simulink model "Approach_Avoid_Task"  (R2019b)
settings: Solver=ode4  StartTime=0.0  StopTime=inf  FixedStep=BKIN_STEP_TIME  RelTol=1e-3  EnableMultiTasking=on
StartFcn:
  |  warndlg('Dexterit-E models cannot run under simulation. Please compile your model and run it from within Dexterit-E.');set_param(bdroot,'SimulationCommand','stop')
model workspace (MAT data in the model file):
  ADJUST_START = 2
  APPROACH_TARGET_COL = 9
  AVOIDVIS_AREA_COL = 3
  AVOID_AREA_COL = 2
  AVOID_DIST_ADJUST = 8
  BEGIN_LABEL_COL = 5
  BEGIN_TARGET_COL = 4
  BKIN_KINEMATIC_FRAME_SIZE = 400
  BKIN_STEP_TIME = 0.00025
  CHECK_ORDER_ACTIVE = 7
  CHECK_ORDER_CIRC = 6
  COLOUR_2ND = 7
  COLOUR_3RD = 11
  COLOUR_4TH = 12
  COLOUR_INIT = 6
  ERROR_DELAY = 12
  ERROR_LABEL_COL = 6
  E_APPROACHED = 19
  E_AVOIDED = 21
  E_BLOCK_1 = 28
  E_BLOCK_2 = 29
  E_BLOCK_3 = 30
  E_BLOCK_4 = 31
  E_ERROR_TRIAL = 23
  E_HAND_IN_START = 17
  E_HAND_LEFT = 16
  E_LEFT_TESTED = 2
  E_LOC_1 = 3
  E_LOC_10 = 12
  E_LOC_11 = 13
  E_LOC_12 = 14
  E_LOC_2 = 4
  E_LOC_3 = 5
  E_LOC_4 = 6
  E_LOC_5 = 7
  E_LOC_6 = 8
  E_LOC_7 = 9
  E_LOC_8 = 10
  E_LOC_9 = 11
  E_NO_EVENT = 0
  E_RIGHT_TESTED = 1
  E_TARGET_ON = 18
  E_TASK_SEQ_1 = 24
  E_TASK_SEQ_2 = 25
  E_TASK_SEQ_3 = 26
  E_TASK_SEQ_4 = 27
  E_TIMED_OUT = 22
  E_TRIAL_END = 20
  E_TRIAL_START = 15
  INFO_TARGET_COL = 8
  LABEL_HEIGHT = 9
  LABEL_TEXT = 8
  LENGTH = 3
  MAX_FORCE = 3
  MAX_FORCE_BG = 4
  NO_SANDWICH = 15
  RADIUS_VIS = 3
  RAMP_DURATION = 5
  RAND_START_DELAY = 10
  REACH_TIME = 13
  SLOW_LABEL_COL = 7
  START_HOLD_DELAY = 9
  START_TARGET_COL = 1
  STROKE_WIDTH = 10
  SUCCESS_DELAY = 11
  TARGET_X = 4
  TARGET_Y = 5
  TARG_DIST = 1
  TARG_LENGTH = 3
  TARG_WIDTH = 4
  TOGGLE_FIELD = 10
  TRIAL_TIME = 14
  WIDTH = 4
  Width = 4
  col_x = 1
  col_y = 2
undefined symbols (not defined in the file): slselsubs
libraries: Video x10, KINARM_EP_loads x5, General x3, KINARM_general x3
settings Model: ModifiedComment=chris -- Wed Feb 16 09:18:30 2005 -- Version 1.1384  ModifiedHistory=Feb 16/05 - Add error repeat, add offset ramp  ExtModeArmWhenConnect=off  ExtModeLogAll=off  OrderedModelArguments=off  Creator=Chris Grebeldinger  LastModifiedBy=User
settings SolverCC: AutoInsertRateTranBlk=on
settings DataIOCC: SaveFormat=Array  SignalLoggingSaveFormat=ModelDataLogs  SaveOutput=off  SaveTime=off  ReturnWorkspaceOutputs=off  SignalLoggingName=sigsOut
settings OptimizationCC: BlockReduction=off  BooleanDataType=off  OptimizeBlockIOStorage=off  BufferReuse=off  GlobalBufferReuse=off  ExpressionFolding=off  ExpressionDepthLimit=2147483647  LocalBlockOutputs=off  InitFltsAndDblsToZero=on  LifeSpan=inf  OptimizeDataStoreBuffers=off  BusAssignmentInplaceUpdate=off
settings DebuggingCC: SaveWithParameterizedLinksMsg=none  UnderspecifiedInitializationDetection=Classic  MergeDetectMultiDrivingBlocksExec=none  SignalResolutionControl=TryResolveAllWithWarning  MultiTaskDSMMsg=warning  FcnCallInpInsideContextMsg=warning  BusObjectLabelMismatch=none  StateNameClashWarn=warning  StrictBusMsg=ErrorOnBusTreatedAsVector  SFUnexpectedBacktrackingDiag=warning  SFNoUnconditionalDefaultTransitionDiag=warning  SFExecutionAtInitializationDiag=none  ArithmeticOperatorsInVariantConditions=warning
settings HardwareCC: ProdBitPerPointer=32  ProdBitPerSizeT=32  ProdBitPerPtrDiffT=32  ProdLargestAtomicFloat=None  ProdWordSize=32  ProdLongLongMode=on  ProdHWDeviceType=Generic->32-bit x86 compatible  TargetLongLongMode=on  TargetIntDivRoundTo=Zero  TargetEndianess=LittleEndian  TargetHWDeviceType=Generic->32-bit x86 compatible
settings ModelReferenceCC: PropagateSignalLabelsOutOfModel=off
settings SFSimCC: SimCustomHeaderCode="#include \"stdlib.h\""  SimUseLocalCustomCode=off  SimParseCustomCode=off  CustomCodeUndefinedFunction=UseInterfaceOnly
settings RTWCC: Description=Simulink Real-Time  SystemTargetFile=slrt.tlc  TemplateMakefile=slrt_default_tmf  RTWUseLocalCustomCode=off  CustomSourceCode="#include \"stdlib.h\""  CodeExecutionProfiling=on
settings CodeAppCC: MaxIdLength=63  StateflowObjectComments=on
settings SimulinkRealTimeCC: TargetFcnLib=ansi_tfl_tmw.mat  GeneratePreprocessorConditionals=Disable all  PreserveStateflowLocalDataDimensions=off
settings ConfigComp: CovMetricSettings=dw  CovHtmlReporting=on  CovSaveCumulativeToWorkspaceVar=on  CovSaveSingleToWorkspaceVar=on  CovExternalEMLEnable=off

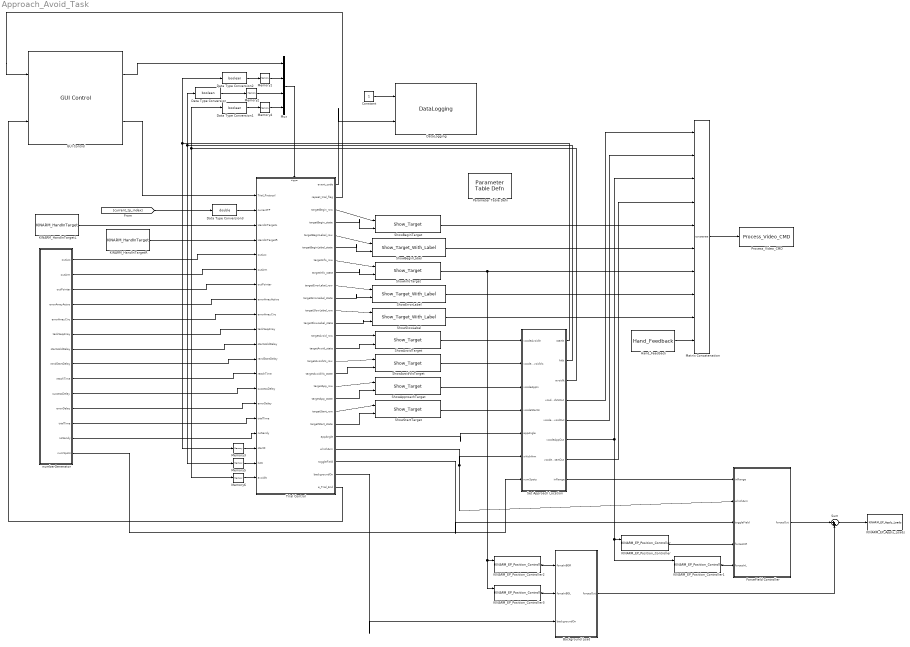
== system Approach_Avoid_Task ==
  Background Load : Subsystem
  Constant : Constant
  Data Type Conversion : DataTypeConversion  OutDataTypeStr=boolean
  Data Type Conversion1 : DataTypeConversion  OutDataTypeStr=boolean
  Data Type Conversion2 : DataTypeConversion  OutDataTypeStr=boolean
  Data Type Conversion3 : DataTypeConversion  OutDataTypeStr=double
  DataLogging : General/DataLogging  log_event_codes=on  log_analog_inputs=off  show_time_remaining=off  ecat_include=on
  ForceField Controller : Subsystem
  GUI Control : General/GUI Control  task_version=1.0  show_repeat_trial_flag=on  use_custom_tp=off  target_type_str=Circle  Target_Type=1  XYcols=[1 2]  Vcols=3  Lcols=4  indices_padding=[0 0 0 0;0 0 0 0]  target_table_rows=64  load_table_rows=20  tp_table_rows=100
  Hand_Feedback : KINARM_general/Hand_Feedback  feedback_cntl_src=none
  KINARM_EP_Apply_Loads : KINARM_EP_loads/KINARM_EP_Apply_Loads  up_duration=1500  down_duration=1500  max_force=30
  KINARM_EP_Position_Controller : KINARM_EP_loads/KINARM_EP_Position_Controller  use_dom_hand=on  inertias_for_FF=KINARM End Point robot  gain_choice=Standard Movement  sample_time=0.001
  KINARM_EP_Position_Controller1 : KINARM_EP_loads/KINARM_EP_Position_Controller  use_dom_hand=off  inertias_for_FF=KINARM End Point robot  gain_choice=Standard Movement  sample_time=0.001
  KINARM_EP_Position_Controller2 : KINARM_EP_loads/KINARM_EP_Position_Controller  use_dom_hand=on  inertias_for_FF=KINARM End Point robot  gain_choice=Standard Movement  sample_time=0.001
  KINARM_EP_Position_Controller3 : KINARM_EP_loads/KINARM_EP_Position_Controller  use_dom_hand=off  inertias_for_FF=KINARM End Point robot  gain_choice=Standard Movement  sample_time=0.001
  KINARM_HandInTargetL : KINARM_general/KINARM_HandInTarget  use_dominant_hand=off  target_type=Circle  num_states=1  attribcol1=[RADIUS_VIS]  attribcol2=[0]  attribcol3=[0]  attribcol4=[0]  attribcol5=[0]
  KINARM_HandInTargetR : KINARM_general/KINARM_HandInTarget  use_dominant_hand=on  target_type=Circle  num_states=1  attribcol1=[RADIUS_VIS]  attribcol2=[0]  attribcol3=[0]  attribcol4=[0]  attribcol5=[0]
  Matrix Concatenation : Concatenate  NumInputs=10  Mode=Multidimensional array
  Memory{1..6} (6 alike) : Memory
  Mux : Mux
  Parameter Table Defn : General/Parameter Table Defn  ShowInLibBrowser=0
  Process_Video_CMD : Video/Process_Video_CMD  video_delay=50
  Set Approach Location : Subsystem
  ShowApproachTarget : Video/Show_Target  target_type=Circle  num_states=1  attribcol1=[COLOUR_INIT 0 0 RADIUS_VIS]  attribcol2=[0 0 0 0]  attribcol3=[0 0 0 0]  attribcol4=[0 0 0 0]  attribcol5=[0 0 0 0]  stateindices_padding=[0 0 0 0 0 0 0;0 0 0 0 0 0 0;0 0 0 0 0 0 0;0 0 0 0 0 0 0;0 0 0 0 0 0 0]  source=dialog  opacity=100  target_display=Both subject and operator displays  num_col=4
  ShowAvoidTarget : Video/Show_Target  target_type=Circle  num_states=1  attribcol1=[COLOUR_INIT COLOUR_2ND STROKE_WIDTH RADIUS_VIS]  attribcol2=[0 0 0 0]  attribcol3=[0 0 0 0]  attribcol4=[0 0 0 0]  attribcol5=[0 0 0 0]  stateindices_padding=[0 0 0 0 0 0 0;0 0 0 0 0 0 0;0 0 0 0 0 0 0;0 0 0 0 0 0 0;0 0 0 0 0 0 0]  source=dialog  opacity=100  target_display=Both subject and operator displays  num_col=4
  ShowAvoidVisTarget : Video/Show_Target  target_type=Circle  num_states=1  attribcol1=[COLOUR_INIT COLOUR_2ND STROKE_WIDTH RADIUS_VIS]  attribcol2=[0 0 0 0]  attribcol3=[0 0 0 0]  attribcol4=[0 0 0 0]  attribcol5=[0 0 0 0]  stateindices_padding=[0 0 0 0 0 0 0;0 0 0 0 0 0 0;0 0 0 0 0 0 0;0 0 0 0 0 0 0;0 0 0 0 0 0 0]  source=dialog  opacity=100  target_display=Both subject and operator displays  num_col=4
  ShowBeginLabel : Video/Show_Target_With_Label  target_type=Circle  num_states=1  attribcol1=[0 0 0 0 LABEL_TEXT COLOUR_2ND LABEL_HEIGHT]  attribcol2=[0 0 0 0 0 0 0]  attribcol3=[0 0 0 0 0 0 0]  attribcol4=[0 0 0 0 0 0 0]  attribcol5=[0 0 0 0 0 0 0]  stateindices_padding=[0 0 0 0;0 0 0 0;0 0 0 0;0 0 0 0;0 0 0 0]  source=dialog  opacity=100  target_display=Both subject and operator displays
  ShowBeginTarget : Video/Show_Target  target_type=Circle  num_states=1  attribcol1=[COLOUR_INIT COLOUR_2ND STROKE_WIDTH RADIUS_VIS]  attribcol2=[0 0 0 0]  attribcol3=[0 0 0 0]  attribcol4=[0 0 0 0]  attribcol5=[0 0 0 0]  stateindices_padding=[0 0 0 0 0 0 0;0 0 0 0 0 0 0;0 0 0 0 0 0 0;0 0 0 0 0 0 0;0 0 0 0 0 0 0]  source=dialog  opacity=100  target_display=Both subject and operator displays  num_col=4
  ShowErrorLabel : Video/Show_Target_With_Label  target_type=Circle  num_states=1  attribcol1=[0 0 0 0 LABEL_TEXT COLOUR_2ND LABEL_HEIGHT]  attribcol2=[0 0 0 0 0 0 0]  attribcol3=[0 0 0 0 0 0 0]  attribcol4=[0 0 0 0 0 0 0]  attribcol5=[0 0 0 0 0 0 0]  stateindices_padding=[0 0 0 0;0 0 0 0;0 0 0 0;0 0 0 0;0 0 0 0]  source=dialog  opacity=100  target_display=Both subject and operator displays
  ShowInfoTarget : Video/Show_Target  target_type=Rectangle  num_states=4  attribcol1=[COLOUR_INIT 0 0 TARGET_X TARGET_Y 0]  attribcol2=[COLOUR_2ND 0 0 TARGET_X TARGET_Y 0]  attribcol3=[COLOUR_3RD 0 0 TARGET_X TARGET_Y 0]  attribcol4=[COLOUR_4TH 0 0 TARGET_X TARGET_Y 0]  attribcol5=[0 0 0 0 0 0]  stateindices_padding=[0 0 0 0 0;0 0 0 0 0;0 0 0 0 0;0 0 0 0 0;0 0 0 0 0]  source=dialog  opacity=100  target_display=Both subject and operator displays  num_col=6
  ShowSlowLabel : Video/Show_Target_With_Label  target_type=Circle  num_states=1  attribcol1=[0 0 0 0 LABEL_TEXT COLOUR_2ND LABEL_HEIGHT]  attribcol2=[0 0 0 0 0 0 0]  attribcol3=[0 0 0 0 0 0 0]  attribcol4=[0 0 0 0 0 0 0]  attribcol5=[0 0 0 0 0 0 0]  stateindices_padding=[0 0 0 0;0 0 0 0;0 0 0 0;0 0 0 0;0 0 0 0]  source=dialog  opacity=100  target_display=Both subject and operator displays
  ShowStartTarget : Video/Show_Target  target_type=Circle  num_states=1  attribcol1=[COLOUR_INIT 0 0 RADIUS_VIS]  attribcol2=[0 0 0 0]  attribcol3=[0 0 0 0]  attribcol4=[0 0 0 0]  attribcol5=[0 0 0 0]  stateindices_padding=[0 0 0 0 0 0 0;0 0 0 0 0 0 0;0 0 0 0 0 0 0;0 0 0 0 0 0 0;0 0 0 0 0 0 0]  source=dialog  opacity=100  target_display=Both subject and operator displays  num_col=4
  Sum : Sum  Inputs=|++
  Trial Control : Stateflow chart  TreatAsAtomicUnit=on
  numberGenerator : Subsystem
  wires:
  Trial Control/25(e_Trial_End) -> GUI Control/2
  Trial Control/20(targetStart_state) -> ShowStartTarget/2
  Trial Control/19(targetStart_row) -> ShowStartTarget/1
  Matrix Concatenation/1 -> Process_Video_CMD/1
  Trial Control/1(event_code) -> DataLogging/2
  ShowStartTarget/1 -> Set Approach Location/4(vcodeStartIn)
  Constant/1 -> DataLogging/1
  GUI Control/2 -> Trial Control/1(Trial_Protocol)
  ForceField Controller/1(forcesOut) -> Sum/1
  Trial Control/17(targetApp_row) -> ShowApproachTarget/1
  Trial Control/18(targetApp_state) -> ShowApproachTarget/2
  Trial Control/15(targetAvoidVis_row) -> ShowAvoidVisTarget/1
  Trial Control/16(targetAvoidVis_state) -> ShowAvoidVisTarget/2
  ShowAvoidVisTarget/1 -> Set Approach Location/2(vcodeAvoidVis)
  Trial Control/2(repeat_trial_flag) -> GUI Control/1
  KINARM_EP_Position_Controller/1 -> ForceField Controller/4(forcesInR)
  GUI Control/1 -> Mux/1
  [current_tp_index] -> Data Type Conversion3/1
  ShowApproachTarget/1 -> Set Approach Location/3(vcodeAppIn)
  Set Approach Location/7(vcodeStartOut) -> Matrix Concatenation/4
  Set Approach Location/6(vcodeAppOut) -> KINARM_EP_Position_Controller1/1, KINARM_EP_Position_Controller/1, Matrix Concatenation/3
  Set Approach Location/5(vcodeAvoidOut) -> Matrix Concatenation/2
  Set Approach Location/1(startIt) -> Data Type Conversion2/1, Memory3/1
  KINARM_EP_Position_Controller1/1 -> ForceField Controller/5(forcesInL)
  numberGenerator/1(outLoc) -> Trial Control/5(outLoc)
  numberGenerator/2(outArm) -> Trial Control/6(outArm)
  Trial Control/21(appAngle) -> Set Approach Location/5(appAngle)
  Trial Control/22(whichArm) -> ForceField Controller/2(whichArm), Set Approach Location/6(whichArm)
  ShowInfoTarget/1 -> KINARM_EP_Position_Controller3/1, KINARM_EP_Position_Controller2/1, Matrix Concatenation/7
  KINARM_HandInTargetR/1 -> Trial Control/4(HandInTargetR)
  KINARM_HandInTargetL/1 -> Trial Control/3(HandInTargetL)
  Trial Control/23(toggleField) -> ForceField Controller/3(toggleField)
  Sum/1 -> KINARM_EP_Apply_Loads/1
  KINARM_EP_Position_Controller2/1 -> Background Load/1(forceInBGR)
  KINARM_EP_Position_Controller3/1 -> Background Load/2(forceInBGL)
  Background Load/1(forcesOut) -> Sum/2
  Trial Control/24(backgroundOn) -> Background Load/3(backgroundOn)
  Trial Control/3(targetBegin_row) -> ShowBeginTarget/1
  Trial Control/4(targetBegin_state) -> ShowBeginTarget/2
  Trial Control/7(targetInfo_row) -> ShowInfoTarget/1
  Trial Control/8(targetInfo_state) -> ShowInfoTarget/2
  Trial Control/5(targetBeginLabel_row) -> ShowBeginLabel/1
  Trial Control/6(targetBeginLabel_state) -> ShowBeginLabel/2
  numberGenerator/3(outPointer) -> Trial Control/7(outPointer)
  Trial Control/9(targetErrorLabel_row) -> ShowErrorLabel/1
  Trial Control/10(targetErrorLabel_state) -> ShowErrorLabel/2
  Trial Control/11(targetSlowLabel_row) -> ShowSlowLabel/1
  Trial Control/12(targetSlowLabel_state) -> ShowSlowLabel/2
  numberGenerator/7(startHoldDelay) -> Trial Control/11(startHoldDelay)
  numberGenerator/14(numSpots) -> Set Approach Location/7(numSpots)
  numberGenerator/5(errorArrayCirc) -> Trial Control/9(errorArrayCirc)
  numberGenerator/4(errorArrayActve) -> Trial Control/8(errorArrayActive)
  numberGenerator/8(randStartDelay) -> Trial Control/12(randStartDelay)
  numberGenerator/12(trialTime) -> Trial Control/16(trialTime)
  numberGenerator/9(reachTime) -> Trial Control/13(reachTime)
  numberGenerator/10(successDelay) -> Trial Control/14(successDelay)
  numberGenerator/11(errorDelay) -> Trial Control/15(errorDelay)
  ShowBeginLabel/1 -> Matrix Concatenation/6
  ShowBeginTarget/1 -> Matrix Concatenation/5
  ShowErrorLabel/1 -> Matrix Concatenation/8
  ShowSlowLabel/1 -> Matrix Concatenation/9
  Hand_Feedback/1 -> Matrix Concatenation/10
  numberGenerator/6(taskSeqArray) -> Trial Control/10(taskSeqArray)
  Set Approach Location/8(inRange) -> ForceField Controller/1(inRange)
  numberGenerator/13(noSandy) -> Trial Control/17(noSandy)
  Memory3/1 -> Trial Control/18(startIt)
  Mux/1 -> Trial Control/Trigger
  Memory2/1 -> Mux/3
  Memory4/1 -> Mux/4
  Set Approach Location/2(hitIt) -> Data Type Conversion/1, Memory5/1
  Set Approach Location/3(avoidIt) -> Memory6/1, Data Type Conversion1/1
  Data Type Conversion/1 -> Memory2/1
  Data Type Conversion1/1 -> Memory4/1
  Data Type Conversion2/1 -> Memory1/1
  Memory1/1 -> Mux/2
  Memory5/1 -> Trial Control/19(hitIt)
  Memory6/1 -> Trial Control/20(avoidIt)
  Data Type Conversion3/1 -> Trial Control/2(currentTP)
  Trial Control/13(targetAvoid_row) -> ShowAvoidTarget/1
  Trial Control/14(targetAvoid_state) -> ShowAvoidTarget/2
  ShowAvoidTarget/1 -> Set Approach Location/1(vcodeAvoidIn)
  Set Approach Location/4(vcodeAvoidVisOut) -> Matrix Concatenation/1

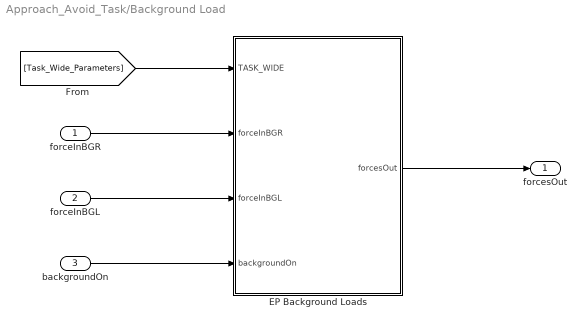
== system Approach_Avoid_Task/Background Load ==
  forceInBGR : Inport
  forceInBGL : Inport  Port=2
  backgroundOn : Inport  Port=3
  EP Background Loads : MATLAB Function  TreatAsAtomicUnit=on
  forcesOut : Outport
  wires:
  [Task_Wide_Parameters] -> EP Background Loads/1(TASK_WIDE)
  EP Background Loads/1(forcesOut) -> forcesOut/1
  forceInBGR/1 -> EP Background Loads/2(forceInBGR)
  forceInBGL/1 -> EP Background Loads/3(forceInBGL)
  backgroundOn/1 -> EP Background Loads/4(backgroundOn)

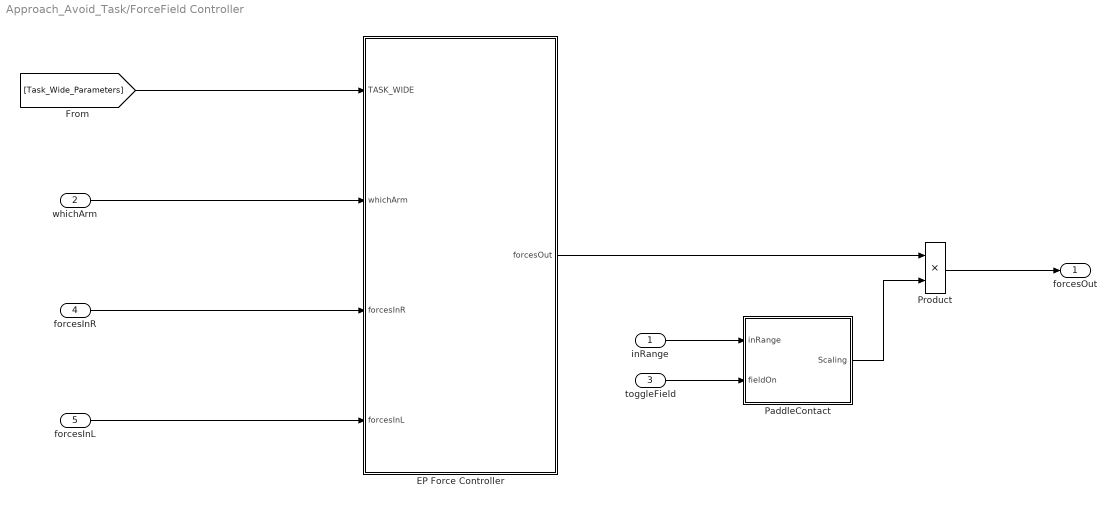
== system Approach_Avoid_Task/ForceField Controller ==
  inRange : Inport
  whichArm : Inport  Port=2
  toggleField : Inport  Port=3
  forcesInR : Inport  Port=4
  forcesInL : Inport  Port=5
  EP Force Controller : MATLAB Function  TreatAsAtomicUnit=on
  PaddleContact : Subsystem  mask(Perturbation){}
  Product : Product
  forcesOut : Outport
  wires:
  [Task_Wide_Parameters] -> EP Force Controller/1(TASK_WIDE)
  EP Force Controller/1(forcesOut) -> Product/1
  toggleField/1 -> PaddleContact/2(fieldOn)
  forcesInR/1 -> EP Force Controller/3(forcesInR)
  whichArm/1 -> EP Force Controller/2(whichArm)
  forcesInL/1 -> EP Force Controller/4(forcesInL)
  PaddleContact/1(Scaling) -> Product/2
  inRange/1 -> PaddleContact/1(inRange)
  Product/1 -> forcesOut/1

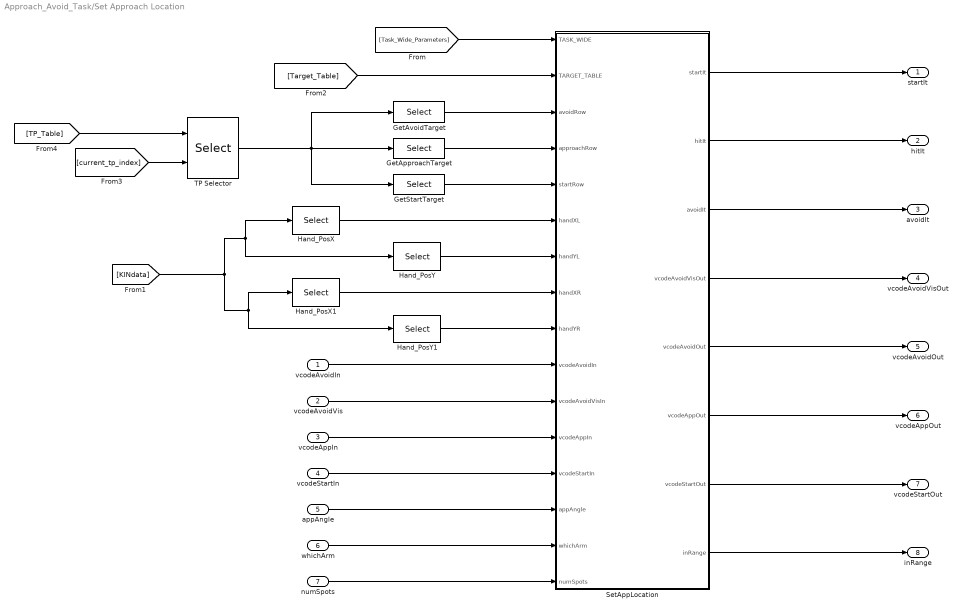
== system Approach_Avoid_Task/Set Approach Location ==
  vcodeAvoidIn : Inport
  vcodeAvoidVis : Inport  Port=2
  vcodeAppIn : Inport  Port=3
  vcodeStartIn : Inport  Port=4
  appAngle : Inport  Port=5
  whichArm : Inport  Port=6
  numSpots : Inport  Port=7
  GetApproachTarget : Selector  NumberOfDimensions=2  InputPortWidth=3  IndexOptions=Select all,Index vector (dialog)  Indices=[1],[APPROACH_TARGET_COL]  OutputSizes=slselsubs([(-2),(-2)],1),slselsubs([(-2),(-2)],2)
  GetAvoidTarget : Selector  NumberOfDimensions=2  InputPortWidth=3  IndexOptions=Select all,Index vector (dialog)  Indices=[1],[AVOID_AREA_COL]  OutputSizes=slselsubs([(-2),(-2)],1),slselsubs([(-2),(-2)],2)
  GetStartTarget : Selector  NumberOfDimensions=2  InputPortWidth=3  IndexOptions=Select all,Index vector (dialog)  Indices=[1],[START_TARGET_COL]  OutputSizes=slselsubs([(-2),(-2)],1),slselsubs([(-2),(-2)],2)
  Hand_PosX : Selector  NumberOfDimensions=2  InputPortWidth=3  IndexOptions=Index vector (dialog),Index vector (dialog)  Indices=[2],[23]  OutputSizes=slselsubs([(-2),(-2)],1),slselsubs([(-2),(-2)],2)
  Hand_PosX1 : Selector  NumberOfDimensions=2  InputPortWidth=3  IndexOptions=Index vector (dialog),Index vector (dialog)  Indices=[1],[23]  OutputSizes=slselsubs([(-2),(-2)],1),slselsubs([(-2),(-2)],2)
  Hand_PosY : Selector  NumberOfDimensions=2  InputPortWidth=3  IndexOptions=Index vector (dialog),Index vector (dialog)  Indices=[2],[24]  OutputSizes=slselsubs([(-2),(-2)],1),slselsubs([(-2),(-2)],2)
  Hand_PosY1 : Selector  NumberOfDimensions=2  InputPortWidth=3  IndexOptions=Index vector (dialog),Index vector (dialog)  Indices=[1],[24]  OutputSizes=slselsubs([(-2),(-2)],1),slselsubs([(-2),(-2)],2)
  SetAppLocation : MATLAB Function  TreatAsAtomicUnit=on
  TP Selector : Selector  NumberOfDimensions=2  InputPortWidth=3  IndexOptions=Index vector (port),Select all  Indices=1,-1  OutputSizes=slselsubs([(-2),(-2)],1),slselsubs([(-2),(-2)],2)
  startIt : Outport
  hitIt : Outport  Port=2
  avoidIt : Outport  Port=3
  vcodeAvoidVisOut : Outport  Port=4
  vcodeAvoidOut : Outport  Port=5
  vcodeAppOut : Outport  Port=6
  vcodeStartOut : Outport  Port=7
  inRange : Outport  Port=8
  wires:
  [Task_Wide_Parameters] -> SetAppLocation/1(TASK_WIDE)
  [current_tp_index] -> TP Selector/2
  Hand_PosX/1 -> SetAppLocation/6(handXL)
  Hand_PosY/1 -> SetAppLocation/7(handYL)
  [TP_Table] -> TP Selector/1
  TP Selector/1 -> GetStartTarget/1, GetApproachTarget/1, GetAvoidTarget/1
  GetApproachTarget/1 -> SetAppLocation/4(approachRow)
  [Target_Table] -> SetAppLocation/2(TARGET_TABLE)
  SetAppLocation/2(hitIt) -> hitIt/1
  vcodeAvoidIn/1 -> SetAppLocation/10(vcodeAvoidIn)
  SetAppLocation/5(vcodeAvoidOut) -> vcodeAvoidOut/1
  vcodeAppIn/1 -> SetAppLocation/12(vcodeAppIn)
  vcodeStartIn/1 -> SetAppLocation/13(vcodeStartIn)
  SetAppLocation/6(vcodeAppOut) -> vcodeAppOut/1
  SetAppLocation/7(vcodeStartOut) -> vcodeStartOut/1
  GetAvoidTarget/1 -> SetAppLocation/3(avoidRow)
  GetStartTarget/1 -> SetAppLocation/5(startRow)
  Hand_PosX1/1 -> SetAppLocation/8(handXR)
  Hand_PosY1/1 -> SetAppLocation/9(handYR)
  [KINdata] -> Hand_PosY/1, Hand_PosX/1, Hand_PosY1/1, Hand_PosX1/1
  SetAppLocation/1(startIt) -> startIt/1
  SetAppLocation/3(avoidIt) -> avoidIt/1
  whichArm/1 -> SetAppLocation/15(whichArm)
  appAngle/1 -> SetAppLocation/14(appAngle)
  numSpots/1 -> SetAppLocation/16(numSpots)
  SetAppLocation/8(inRange) -> inRange/1
  vcodeAvoidVis/1 -> SetAppLocation/11(vcodeAvoidVisIn)
  SetAppLocation/4(vcodeAvoidVisOut) -> vcodeAvoidVisOut/1

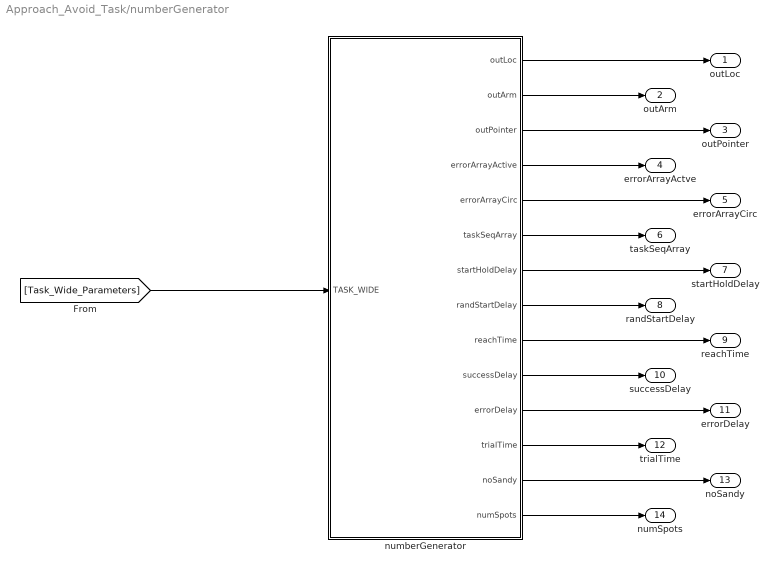
== system Approach_Avoid_Task/numberGenerator ==
  numberGenerator : MATLAB Function  TreatAsAtomicUnit=on
  outLoc : Outport
  outArm : Outport  Port=2
  outPointer : Outport  Port=3
  errorArrayActve : Outport  Port=4
  errorArrayCirc : Outport  Port=5
  taskSeqArray : Outport  Port=6
  startHoldDelay : Outport  Port=7
  randStartDelay : Outport  Port=8
  reachTime : Outport  Port=9
  successDelay : Outport  Port=10
  errorDelay : Outport  Port=11
  trialTime : Outport  Port=12
  noSandy : Outport  Port=13
  numSpots : Outport  Port=14
  wires:
  numberGenerator/1(outLoc) -> outLoc/1
  numberGenerator/2(outArm) -> outArm/1
  numberGenerator/5(errorArrayCirc) -> errorArrayCirc/1
  numberGenerator/3(outPointer) -> outPointer/1
  [Task_Wide_Parameters] -> numberGenerator/1(TASK_WIDE)
  numberGenerator/4(errorArrayActive) -> errorArrayActve/1
  numberGenerator/14(numSpots) -> numSpots/1
  numberGenerator/7(startHoldDelay) -> startHoldDelay/1
  numberGenerator/8(randStartDelay) -> randStartDelay/1
  numberGenerator/12(trialTime) -> trialTime/1
  numberGenerator/9(reachTime) -> reachTime/1
  numberGenerator/10(successDelay) -> successDelay/1
  numberGenerator/11(errorDelay) -> errorDelay/1
  numberGenerator/6(taskSeqArray) -> taskSeqArray/1
  numberGenerator/13(noSandy) -> noSandy/1

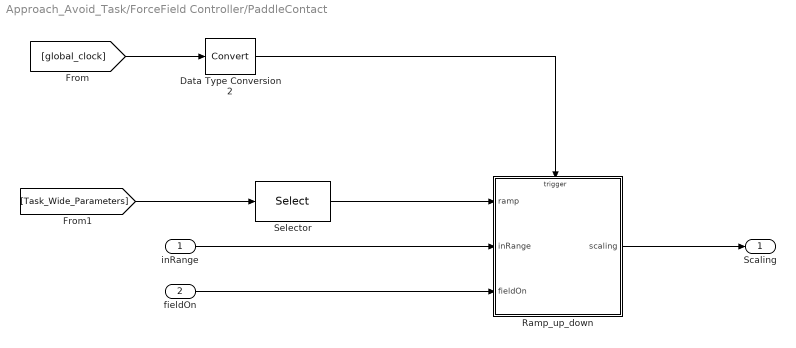
== system Approach_Avoid_Task/ForceField Controller/PaddleContact ==
  inRange : Inport
  fieldOn : Inport  Port=2
  Data Type Conversion2 : DataTypeConversion
  Ramp_up_down : Stateflow chart  TreatAsAtomicUnit=on
  Selector : Selector  NumberOfDimensions=2  InputPortWidth=3  IndexOptions=Index vector (dialog),Select all  Indices=[RAMP_DURATION],[3]  OutputSizes=slselsubs([(-2),(-2)],1),1
  Scaling : Outport
  wires:
  Ramp_up_down/1(scaling) -> Scaling/1
  [global_clock] -> Data Type Conversion2/1
  Data Type Conversion2/1 -> Ramp_up_down/Trigger
  [Task_Wide_Parameters] -> Selector/1
  Selector/1 -> Ramp_up_down/1(ramp)
  inRange/1 -> Ramp_up_down/2(inRange)
  fieldOn/1 -> Ramp_up_down/3(fieldOn)

== matlab function Approach_Avoid_Task/Set Approach Location/SetAppLocation ==
  data: startIt output; hitIt output; avoidIt output; vcodeAvoidVisOut output; vcodeAvoidOut output; vcodeAppOut output; vcodeStartOut output; TASK_WIDE input; TARGET_TABLE input; avoidRow input; approachRow input; startRow input; handXL input; handYL input; handXR input; handYR input; vcodeAvoidIn input; vcodeAvoidVisIn input; vcodeAppIn input; vcodeStartIn input; appAngle input; whichArm input; numSpots input; TARG_DIST parameter; RADIUS_VIS parameter; ADJUST_START parameter; TARGET_X parameter; TARGET_Y parameter; inRange output; AVOID_DIST_ADJUST parameter
function [startIt, hitIt, avoidIt, vcodeAvoidVisOut, vcodeAvoidOut, vcodeAppOut, vcodeStartOut, inRange] = fcn...
    (TASK_WIDE, TARGET_TABLE, avoidRow, approachRow, startRow, handXL, handYL, handXR, handYR, vcodeAvoidIn, vcodeAvoidVisIn, vcodeAppIn, vcodeStartIn, appAngle, whichArm, numSpots,...
    TARG_DIST, RADIUS_VIS, ADJUST_START, TARGET_X, TARGET_Y, AVOID_DIST_ADJUST)
%This function checks if the hand is in start, approach or avoid targets.

%% initialize hand and location to be displayed
targDist = TASK_WIDE(TARG_DIST); %gets distance of targets set from task wide
adjustStart = TASK_WIDE(ADJUST_START); %adjusts the left and right distance from the midline for the center of start/approach/avoid targets
avoidDistAdjust = TASK_WIDE(AVOID_DIST_ADJUST)/100;
angleArray = [0:2*pi/numSpots:2*pi-2*pi/numSpots]; %get radians for each location

%assume hand is right hand being tested
handX = handXR;
handY = handYR;
whichLoc = angleArray(appAngle); %get the location

if (whichArm == 1) %1 is left arm, left arm is being tested
	adjustStart = -TASK_WIDE(ADJUST_START); %shift target center to the left
    handX = handXL;
    handY = handYL;
end

%% initialize radius

rValStart = TARGET_TABLE(startRow,RADIUS_VIS)*0.01; %radius of start target
rValApp = TARGET_TABLE(approachRow,RADIUS_VIS)*0.01; %radius of approach target
rValApp2 = targDist*0.01-rValStart; %radius of force field around approach target accounts for starting target
rValAvoid = TARGET_TABLE(avoidRow,RADIUS_VIS)*0.01; %radius of avoid target

%% change vcodes for start target contact
%Checks if hand is inside of start target (circle) and shamelessly stolen 
%from HandInTarget block and simplified.
vcodeStartOut = vcodeStartIn;

vcodeStartOut(3) = vcodeStartIn(3) + adjustStart*0.01; %x position adjusted depending on arm assessed
vcodeStartOut(4) = vcodeStartIn(4);

deltaxStart=handX-vcodeStartOut(3); %find difference between hand and approach target
deltayStart=handY-vcodeStartOut(4);

distanceStart = deltaxStart.^2 + deltayStart.^2;
if (distanceStart <= rValStart.^2) %if hand is in start target then trigger start
    startIt = 1;
else
    startIt = 0;
end

%% change vcodes for approach target contact
%Same as above but for approach target (circle).
vcodeAppOut = vcodeAppIn;

vcodeAppOut(3) = vcodeAppIn(3) + targDist*cos(whichLoc)*0.01 + adjustStart*0.01;
vcodeAppOut(4) = vcodeAppIn(4) + targDist*sin(whichLoc)*0.01;

deltaxApp=handX-vcodeAppOut(3);
deltayApp=handY-vcodeAppOut(4);

distanceApp = deltaxApp.^2 + deltayApp.^2;
if (distanceApp < rValApp.^2) %if hand inside approach target
    hitIt = 1;
else
    hitIt = 0;
end

if (distanceApp < rValApp2.^2) %if hand inside approach target force field
    inRange = 1;
else
    inRange = 0;
end

% used when target was a rectangle, now it is a circle
% xLength = TARGET_TABLE(approachRow,TARGET_X)*0.01;  %width (sizes in cm in v1.4)
% yLength = TARGET_TABLE(approachRow,TARGET_Y)*0.01;  %height (sizes in cm in v1.4)

% if (abs(deltax) <= xLength/2 && abs(deltay) <= yLength/2) %if hand is inside any part of the rectangle then trigger hit
%     e_hit = 1;
% else
%     e_hit = 0;
% end
% 
% if (abs(deltax2) <= xLength/2 && abs(deltay2) <= yLength/2) %if hand is inside any part of the rectangle then trigger hit
%     handInRange = 1;
% else
%     handInRange = 0;
% end

%% change vcodes for avoid target no contact
%similar to above but checks if hand is inside avoid target (circle)
% vcodeAvoidOut = vcodeAvoidIn;
% 
% vcodeAvoidOut(3) = (vcodeAvoidIn(3) + targDist*cos(whichLoc+pi)*0.01*avoidDistAdjust + adjustStart*0.01);
% vcodeAvoidOut(4) = (vcodeAvoidIn(4) + targDist*sin(whichLoc+pi)*0.01*avoidDistAdjust);
% vcodeAvoidOut(12) = whichLoc+pi;
% 
% deltaxAvoid=handX-vcodeAvoidOut(3);
% deltayAvoid=handY-vcodeAvoidOut(4);
% 
% cosAngle = cos(vcodeAvoidOut(12));
% sinAngle = sin(vcodeAvoidOut(12));
% 
% xrotate=deltaxAvoid.*cosAngle + deltayAvoid.*sinAngle;   %location of x point in rectangle's coordinate frame
% yrotate=-deltaxAvoid.*sinAngle + deltayAvoid.*cosAngle;  %location of y point in rectangle's coordinate frame
% 
% xLength = TARGET_TABLE(avoidRow,TARGET_X)*0.01;  %width (sizes in cm in v1.4)
% yLength = TARGET_TABLE(avoidRow,TARGET_Y)*0.01;
% 
% if (abs(xrotate) <= xLength/2 && abs(yrotate) <= yLength/2)
%     avoidIt = 1;
% else
%     avoidIt = 0;
% end

vcodeAvoidOut = vcodeAvoidIn;

vcodeAvoidOut(3) = vcodeAvoidIn(3) + targDist*cos(whichLoc+pi)*0.01 + adjustStart*0.01;
vcodeAvoidOut(4) = vcodeAvoidIn(4) + targDist*sin(whichLoc+pi)*0.01;

deltaxAvoid=handX-vcodeAvoidOut(3);
deltayAvoid=handY-vcodeAvoidOut(4);

distanceAvoid = deltaxAvoid.^2 + deltayAvoid.^2;
if (distanceAvoid < rValAvoid.^2) %if hand inside approach target
    avoidIt = 1;
else
    avoidIt = 0;
end
 
% distanceAvoid = deltaxAvoid.^2 + deltayAvoid.^2;
% if (distanceAvoid < rValAvoid.^2) %if hand outside of avoid target then send avoid trigger
%     avoidIt = 1;
% else
%     avoidIt = 0;
% end

%% change vcodes for avoid target no contact
%similar to above but checks if hand is outside avoid target (circle)
vcodeAvoidVisOut = vcodeAvoidVisIn;

vcodeAvoidVisOut(3) = vcodeAvoidVisIn(3) + adjustStart*0.01;
vcodeAvoidVisOut(4) = vcodeAvoidVisIn(4);

== stateflow chart Approach_Avoid_Task/Trial Control ==
  state Initialize/
    %Task checks if the participant reached for a certain trial or avoided
    %a certain trial successfully,
    %Starts from block type A, switches to type B, continues B, then
    %switch back to block A. A and B can be circle/square or
    %active/sedentary blocks
    %Added functionality to automize block switching
    %set rows for start, approach, avoid targets and relevant times
    entry:
    targetStart_state = 0;
    targetApp_state = 0;
    targetAvoid_state = 0;
    targetInfo_row = Trial_Protocol(INFO_TARGET_COL);
    targetBegin_row = Trial_Protocol(BEGIN_TARGET_COL);
    targetBeginLabel_row = Trial_Protocol(BEGIN_LABEL_COL);
    targetErrorLabel_row = Trial_Protocol(ERROR_LABEL_COL);
    targetStart_row = Trial_Protocol(START_TARGET_COL);
    targetAvoidVis_row = Trial_Protocol(AVOIDVIS_AREA_COL);
    targetErrorLabel_state = 0;
    targetSlowLabel_row = Trial_Protocol(SLOW_LABEL_COL);
    targetSlowLabel_state = 0;
    targetInfo_state = 0;
    trialCount = 1;
    backgroundOn = 0;
    tpCount = zeros(1,24);
    blockCount = 0;
    checkSandwich = noSandy;
  state MainTrial
    state StartofTrial/
      % Turn on starting target.
      entry:
      event_code = E_TRIAL_START;
      targetApp_row = Trial_Protocol(APPROACH_TARGET_COL);
      targetAvoid_row = Trial_Protocol(AVOID_AREA_COL);
      holdStartTime = startHoldDelay + rand()*randStartDelay;
      targetStart_state = 1;
      targetApp_state = 0;
      targetAvoid_state = 0;
      targetAvoidVis_state = 1;
      toggleField = 0;
      repeat_trial_flag = 0;
      tpCount(currentTP) = tpCount(currentTP) + 1;
      pointer = outPointer(tpCount(currentTP),currentTP);
      appAngle = outLoc(pointer);
      whichArm = outArm(pointer);
    state outputBlockOrder/
      %indicate the order of blocks
      entry:
      taskSeq = mod(currentTP,4)+1;
      event_code = 23 + taskSeq;
    state setCircle/
      %set circle/square block array
      entry:
      testArray = taskSeqArray(taskSeq,97:192);
    state BeginTask/
      % Turn off begin targets
      entry:
      targetBegin_state = 0;
      targetBeginLabel_state = 0;
      targetInfo_state = 0;
      backgroundOn = 1;
    state skipSandwich/
      %remove sandwich block order
      entry:
      blockCount = 4;
    state setActive/
      %set active/sedentary block array
      entry:
      testArray = taskSeqArray(taskSeq,1:96);
    state thirdBlock/
      %readjust trialCount
      entry:
      trialCount = 49;
    state beginState/
      %show beginning targets
      entry:
      targetBegin_state = 1;
      targetBeginLabel_state = 1;
      blockCount = blockCount + 1;
      event_code = blockCount + 27;
    state HandInStart/
      % Hold hand at start target
      entry:
      event_code = E_HAND_IN_START;
    state handLeft/
      entry:
      event_code = E_HAND_LEFT;
    state firstBlock/
      %reset trialCount
      entry:
      trialCount = 1;
    state setCircleAvoid/
      %show image of circle avoid
      entry:
      targetInfo_state = 4;
    state setCircleApproach/
      %show image of circle approach
      entry:
      targetInfo_state = 3;
    state setActiveAvoid/
      %show image of active avoid
      entry:
      targetInfo_state = 2;
    state tpIndexer/
      entry:
      event_code = 2 + appAngle;
    state setActiveApproach/
      %show image of active approach
      entry:
      targetInfo_state = 1;
    state sayArm/
      entry:
      event_code = 1 + whichArm;
    state Approached/
      %hand is in approach
      entry:
      event_code = E_APPROACHED;
      toggleField = 0;
    state AppOn/
      % Turn on approach target and turn
      %on toggle field if necessary
      entry:
      event_code = E_TARGET_ON;
      toggleField = Trial_Protocol(TOGGLE_FIELD);
      targetStart_state = 0;
      targetApp_state = 1;
      targetAvoid_state = 1;
    state Avoided/
      %hand left avoid target
      entry:
      event_code = E_AVOIDED;
      toggleField = 0;
    state checkError/
      %send out an error for being bad
      entry:
      event_code = E_ERROR_TRIAL;
      targetErrorLabel_state = 1;
    state TimedOut/
      %too slow to reach start/app/avoid
      entry:
      event_code = E_TIMED_OUT;
      targetSlowLabel_state = 1;
      toggleField = 0;
    state EndOfTrial/
      % Turn off targets,
      entry:
      targetStart_state = 0;
      targetAvoid_state = 0;
      targetApp_state = 0;
      toggleField = 0;
      targetAvoidVis_state = 1;
    (junction 226) -> setCircle [order 1] : %if circle or square block
        | [currentTP > 12]
    outputBlockOrder -> (junction 226) : after(5,msec)
    setCircle -> setCircleApproach [order 1] : %circle approach block
        | [testArray(trialCount) == 1]
    setCircle -> setCircleAvoid [order 2] : %circle avoid block
        | [testArray(trialCount) == 0]
    BeginTask -> StartofTrial
    skipSandwich -> (junction 226)
    beginState -> BeginTask [order 1] : %if left hand is in begin target
        | [HandInTargetL(targetBegin_row) == 1]
    beginState -> BeginTask [order 2] : %if right hand is in begin target
        | [HandInTargetR(targetBegin_row) == 1]
    (junction 226) -> setActive [order 2] : %if active or sedentary block
        | [currentTP < 13]
    (junction 226) -> (junction 295) [order 3]
    thirdBlock -> (junction 226)
    firstBlock -> (junction 226)
    (junction 233) -> (junction 226) [order 3] : %contrinued block type
        | [blockCount == 2]
    StartofTrial -> TimedOut [order 1] : %delay after not starting
        | after(trialTime, msec)
    StartofTrial -> (junction 299) [order 2] : after(2,msec)
    setActive -> setActiveApproach [order 2] : %approach active block
        | [testArray(trialCount) == 1]
    setActive -> setActiveAvoid [order 1] : %avoid active block
        | [testArray(trialCount) == 0]
    handLeft -> (junction 299) : after(2,msec)
    (junction 299) -> HandInStart : %checks if hand is
        | %in start
        | [startIt == 1]
    (junction 233) -> thirdBlock [order 1] : %switched block type
        | [blockCount == 3]
    setCircleAvoid -> beginState
    (junction 233) -> firstBlock [order 2] : %switched block type
        | [blockCount == 1]
    (junction 301) -> handLeft [order 1] : %check if hand left
        | [startIt == 0]
    HandInStart -> (junction 301) : %delay after hand in target
        | after(holdStartTime, msec)
    setActiveApproach -> beginState
    setActiveAvoid -> beginState
    setCircleApproach -> beginState
    (junction 301) -> tpIndexer [order 2] : %check if hand is still in
        | [startIt == 1]
    tpIndexer -> sayArm : %delay to write event code
        | after(2,msec)
    sayArm -> AppOn : %delay to write event code
        | after(2,msec)
    Approached -> checkError [order 1] : %if sedentary or square trial and goal is to avoid
        | [((currentTP>6 && currentTP<13) || (currentTP >18)) && testArray(trialCount) == 1]
    AppOn -> Approached [order 1] : %check if either edge hit
        | e_hit
    AppOn -> Approached [order 4] : %would be using just this
        | %but i get an error without
        | %the trigger
        | [hitIt == 1]
    Approached -> checkError [order 3] : %if active or circle trial and goal is to avoid
        | [((currentTP<7) || (currentTP > 12 && currentTP < 19)) && testArray(trialCount) == 0]
    Approached -> EndOfTrial [order 2] : %delay after successful trial
        | after(successDelay,msec)
    AppOn -> Avoided [order 2] : %check if either edge avoid
        | e_avoid
    AppOn -> Avoided [order 5] : %same logic as
        | %start or hit
        | [avoidIt == 1]
    AppOn -> TimedOut [order 3] : %delay after not reaching
        | after(reachTime, msec)
    Avoided -> checkError [order 1] : %if sedentary or square trial and goal is to approach
        | [((currentTP>6 && currentTP<13) || (currentTP >18)) && testArray(trialCount) == 0]
    Avoided -> checkError [order 3] : %if active or circle trial and goal is to approach
        | [((currentTP<7) || (currentTP > 12 && currentTP < 19)) && testArray(trialCount) == 1]
    Avoided -> EndOfTrial [order 2] : %delay after successful trial
        | after(successDelay,msec)
    checkError -> EndOfTrial : %delay after error trial
        | after(errorDelay,msec)
    TimedOut -> EndOfTrial : %delay after error trial
        | after(errorDelay,msec)
  state Inter_Trial_State/
    % Turn off targets, reset the event code, and send the
    %e_Trial_End Stateflow event to indicate that the trial is over.
    entry:
    event_code = 0;
    toggleField = 0;
    targetApp_state = 0;
    targetStart_state = 0;
    targetAvoid_state = 0;
    repeat_trial_flag = 0;
    targetSlowLabel_state = 0;
    targetErrorLabel_state = 0;
    trialCount = trialCount + 1;
    e_Trial_End;
  state RepeatTrial/
    entry:
    repeat_trial_flag = 1;
  (junction 173) -> StartofTrial [order 5] : %keep the trials flowing if the block hasn't ended
  (default) -> Initialize
  Initialize -> outputBlockOrder [order 2] : %wait for task to start
      | [currentTP > 0]
  Initialize -> skipSandwich [order 1] : %check if sandwich block and wait for task to start
      | [checkSandwich == 1 && currentTP > 0]
  (junction 173) -> (junction 226) [order 4] : %event codes for blocks will be unnamed past 4
      | %if past 4 blocks and finished first of block pair (odd block)
      | [mod((trialCount-1),48) == 0 && blockCount > 4 && mod(blockCount,2) == 1]
  (junction 173) -> firstBlock [order 1] : %event codes for blocks will be unnamed past 4
      | %if past 4 blocks and end of block pair (even block)
      | [mod((trialCount-1),96) == 0 && blockCount > 4 && mod(blockCount,2) == 0]
  (junction 173) -> firstBlock [order 3] : %at the end of sandwich blocks, reset trials and continue if more blocks
      | [mod((trialCount-1),96) == 0 && blockCount == 4]
  (junction 173) -> (junction 233) [order 2] : %check if end of block
      | [mod((trialCount-1),48) == 0 && blockCount < 4]
  Inter_Trial_State -> (junction 173) : %arbitrary delay
      | after(errorDelay,msec)
  RepeatTrial -> Inter_Trial_State : after(1,msec)
  MainTrial -> RepeatTrial : e_ExitTrialNow/
      | {tickCount = 1;}
      | % e_ExitTrialNow event occurs if the
      | % Dex pause is pressed by the operator
  EndOfTrial -> Inter_Trial_State : after(1, msec)
  data: event_code output double [0..]; repeat_trial_flag output; targetBegin_row output; targetBegin_state output; targetBeginLabel_row output; targetBeginLabel_state output; targetInfo_row output; targetInfo_state output; targetErrorLabel_row output; targetErrorLabel_state output; targetSlowLabel_row output; targetSlowLabel_state output; targetAvoid_row output; targetAvoid_state output; targetAvoidVis_row output; targetAvoidVis_state output; targetApp_row output [1..32]; targetApp_state output double; targetStart_row output; targetStart_state output; appAngle output; whichArm output; tickCount local double; Trial_Protocol input double; toggleField output; currentTP input; HandInTargetL input; HandInTargetR input; outLoc input; outArm input; outPointer input; errorArrayActive input; errorArrayCirc input; taskSeqArray input; startHoldDelay input; backgroundOn output; pointer local; randStartDelay input; numSpots local; trialCount local; tpCount local; testArray local; blockCount local; reachTime input; successDelay input; errorDelay input; trialTime input; noSandy input; holdStartTime local; startIt input; checkSandwich local; hitIt input; avoidIt input; taskSeq local
  data targetApp_row settings: description=index of the row currently being used in the TargetTable
  events: e_clk input RISING_EDGE_EVENT; e_ExitTrialNow input EITHER_EDGE_EVENT; e_start input EITHER_EDGE_EVENT; e_Trial_End output EITHER_EDGE_EVENT; e_hit input EITHER_EDGE_EVENT; e_avoid input EITHER_EDGE_EVENT

== matlab function Approach_Avoid_Task/ForceField Controller/EP Force Controller ==
  data: TASK_WIDE input; whichArm input; MAX_FORCE parameter; forcesInR input; forcesInL input; forcesOut output
function forcesOut  = fcn(TASK_WIDE, whichArm, MAX_FORCE, forcesInR, forcesInL)
%Function applies a load to the arm when the hand leaves the start target
%and the trial is a loaded trial (toggleField == 1).

%% initialize
maxForce = TASK_WIDE(MAX_FORCE);

if (whichArm == 1)
    forcesIn = forcesInL;
else
    forcesIn = forcesInR;
end

%% set forces out
%Send out forces to the appropriate arm also shamelessly stolen.

posCon_force1 = sqrt(forcesIn(1)^2 + forcesIn(2)^2);
posCon_force2 = sqrt(forcesIn(3)^2 + forcesIn(4)^2);

forcesOut = -forcesIn;
% limit the force of arm 1
if posCon_force1 > maxForce
    scaling = maxForce / posCon_force1;
    forcesOut(1:2) = forcesOut(1:2) * scaling;
end

% limit the force of arm 2
if posCon_force2 > maxForce
    scaling = maxForce / posCon_force2;
    forcesOut(3:4) = forcesOut(3:4) * scaling;
end

== matlab function Approach_Avoid_Task/numberGenerator/numberGenerator ==
  data: TASK_WIDE input; outLoc output; outArm output; outPointer output; errorArrayActive output; errorArrayCirc output; taskSeqArray output; startHoldDelay output; randStartDelay output; reachTime output; successDelay output; errorDelay output; trialTime output; noSandy output; numSpots output; CHECK_ORDER_CIRC parameter; CHECK_ORDER_ACTIVE parameter; START_HOLD_DELAY parameter; RAND_START_DELAY parameter; REACH_TIME parameter; TRIAL_TIME parameter; SUCCESS_DELAY parameter; ERROR_DELAY parameter; NO_SANDWICH parameter
function [outLoc, outArm, outPointer, errorArrayActive, errorArrayCirc, taskSeqArray, startHoldDelay, randStartDelay, reachTime, successDelay, errorDelay, trialTime, noSandy, numSpots] =...
    fcn(TASK_WIDE, CHECK_ORDER_CIRC, CHECK_ORDER_ACTIVE, START_HOLD_DELAY, RAND_START_DELAY, REACH_TIME, TRIAL_TIME, SUCCESS_DELAY, ERROR_DELAY, NO_SANDWICH)  
%This function sets up the random numbers used to guide the location and
%arms tested (numSpots must be set to 12 and numRows needs to be big, i 
%think 128 is fine)
%This function also calls task wide parameters to be used in the trial
%control

%% set up random arrays for location and arm
%Random arrays are generated that put each of the approach and avoid
%targets in one of 12 locations for each arm.
%Lots of work was done so that each location and arm has at least 1
%approach and 1 avoid trial.
numSpots = 12;
numRows = 16;

persistent atTime0 randPointer randTempH randTempL randTempH2 randTempL2 randArm randLoc randSetup
if (isempty(atTime0))
    atTime0 = 0;
    randPointer = zeros(numRows,numSpots*2); %array that gets tp and points to specific location and arm combination
    randArm = [zeros(1,numSpots) ones(1,numSpots)]; %array that account for left and right arms (1 = left arm, 0 = right arm)
    randLoc = [1:numSpots,1:numSpots]; %array that accounts for each location (1-12) where east is 1 and proceeds counterclockwise
    randTempH = zeros(numRows,numSpots*2); %the next bit is a bunch of random generation that I think is necessary but might not be
    randTempL = zeros(numRows,numSpots*2);
    randTempH2 = zeros(numRows,numSpots*2);
    randTempL2 = zeros(numRows,numSpots*2);
    for (i = 1:numRows)
        randTempH(i,:) = [randperm(numSpots*2)];
        randTempL(i,:) = [randperm(numSpots*2)];
        randTempH2(i,:) = [randperm(numSpots*2)];
        randTempL2(i,:) = [randperm(numSpots*2)];
    end
    for (i = 1:4:numRows) %set up pointer array to account for each location,arm,approach/avoid target
        randPointer(i,:) = [randTempH(i,1:numSpots/2) randTempL(i,1:numSpots/2) randTempH2(i,1:numSpots/2) randTempL2(i,1:numSpots/2)];
        randPointer(i+1,:) = [randTempH(i,1+numSpots/2:numSpots) randTempL(i,1+numSpots/2:numSpots) randTempH2(i,1+numSpots/2:numSpots) randTempL2(i,1+numSpots/2:numSpots)];
        randPointer(i+2,:) = [randTempH(i,1+numSpots:numSpots+numSpots/2) randTempL(i,1+numSpots:numSpots+numSpots/2) randTempH2(i,1+numSpots:numSpots+numSpots/2) randTempL2(i,1+numSpots:numSpots+numSpots/2)];
        randPointer(i+3,:) = [randTempH(i,1+numSpots+numSpots/2:numSpots*2) randTempL(i,1+numSpots+numSpots/2:numSpots*2) randTempH2(i,1+numSpots+numSpots/2:numSpots*2) randTempL2(i,1+numSpots+numSpots/2:numSpots*2)];
    end
end

outLoc = randLoc;
outArm = randArm;
outPointer = randPointer;

%% get the task sequence
%Made a feature that lets the person select whether active/sedentary or
%circle/square are approach or avoid first

checkOrderActive = TASK_WIDE(CHECK_ORDER_ACTIVE);
checkOrderCirc = TASK_WIDE(CHECK_ORDER_CIRC);

% if (randSetup == 1)
%     errorArrayActive = [ones(1,numSpots*4) zeros(1,numSpots*4)];
%     errorArrayCirc = [ones(1,numSpots*4) zeros(1,numSpots*4)];
% elseif (randSetup == 2)
%     errorArrayActive = [ones(1,numSpots*4) zeros(1,numSpots*4)];
%     errorArrayCirc = [zeros(1,numSpots*4) ones(1,numSpots*4)];
% elseif (randSetup == 3)
%     errorArrayActive = [zeros(1,numSpots*4) ones(1,numSpots*4) ];
%     errorArrayCirc = [ones(1,numSpots*4) zeros(1,numSpots*4)];
% else
%     errorArrayActive = [zeros(1,numSpots*4) ones(1,numSpots*4)];
%     errorArrayCirc = [zeros(1,numSpots*4) ones(1,numSpots*4)];
% end
errorArrayActive = 1; %unused but kept just in case
errorArrayCirc = 1;

taskSeqArray = [[ones(1,numSpots*4) zeros(1,numSpots*4)], [ones(1,numSpots*4) zeros(1,numSpots*4)];
                [ones(1,numSpots*4) zeros(1,numSpots*4)], [zeros(1,numSpots*4) ones(1,numSpots*4)];
                [zeros(1,numSpots*4) ones(1,numSpots*4)], [ones(1,numSpots*4) zeros(1,numSpots*4)];
                [zeros(1,numSpots*4) ones(1,numSpots*4)], [zeros(1,numSpots*4) ones(1,numSpots*4)]];

used = 1;
if (used == 0)
    if (checkOrderActive == 1) %1 means active approach condition first then active avoid
        errorArrayActive = [ones(1,numSpots*4) zeros(1,numSpots*4)];
    else %0 is the other way
        errorArrayActive = [zeros(1,numSpots*4) ones(1,numSpots*4)];
    end

    if (checkOrderCirc == 1) %1 means circle approach condition first then square avoid
        errorArrayCirc = [ones(1,numSpots*4) zeros(1,numSpots*4)];
    else %0 is the other way
        errorArrayCirc = [zeros(1,numSpots*4) ones(1,numSpots*4)];
    end
end

%% task wide parameter outputs
startHoldDelay = TASK_WIDE(START_HOLD_DELAY);
randStartDelay = TASK_WIDE(RAND_START_DELAY);
trialTime = TASK_WIDE(TRIAL_TIME);
successDelay = TASK_WIDE(SUCCESS_DELAY);
errorDelay = TASK_WIDE(ERROR_DELAY);
reachTime = TASK_WIDE(REACH_TIME);
noSandy = TASK_WIDE(NO_SANDWICH);

== matlab function Approach_Avoid_Task/Background Load/EP Background Loads ==
  data: TASK_WIDE input; forcesOut output; forceInBGR input; forceInBGL input; backgroundOn input; MAX_FORCE_BG parameter
function forcesOut  = fcn(TASK_WIDE, forceInBGR, forceInBGL, backgroundOn, MAX_FORCE_BG)
%Function applies a background load to both arms towards the midline.

%% initialize
forcesOut = zeros(1,4);
maxForceBG = TASK_WIDE(MAX_FORCE_BG);

%% set forces
posCon_force1BG = sqrt(forceInBGR(1)^2 + forceInBGR(2)^2);
posCon_force2BG = sqrt(forceInBGL(3)^2 + forceInBGL(4)^2);

if (backgroundOn == 1)
    % limit the force of arm 1
    if posCon_force1BG > maxForceBG
        scaling = maxForceBG / posCon_force1BG;
        forcesOut(1:2) = forceInBGR(1:2) * scaling;
    end

    % limit the force of arm 2
    if posCon_force2BG > maxForceBG
        scaling = maxForceBG / posCon_force2BG;
        forcesOut(3:4) = forceInBGL(3:4) * scaling;
    end
end

== stateflow chart Approach_Avoid_Task/ForceField Controller/PaddleContact/Ramp_up_down ==
  state peak/
    entry:
    scaling=1;
  state RampingUp/
    %sigmoidal ramping taken from Ethan Heming and
    %modified by Kayne
    entry:
    tick=0;
    CurrScale=scaling;
    b=ramp/4; % Center at Middle;
    c=ramp/20; % Define Rise Rate;
    during:
    tick++;
    scaling = (1-CurrScale)/(1+exp(-1*(tick-b)/c))+CurrScale;
  state RampingDown/
    entry:
    tick=0;
    CurrScale=scaling;
    b=ramp/4; % Center at Middle;
    c=ramp/20; % Define Drop Rate;
    during:
    tick++;
    scaling = CurrScale*(1-1/(1+exp(-1*(tick-b)/c)));
  state minimum/
    entry:
    scaling=0;
  peak -> RampingDown [order 1] : %check if forcefield is turned off
      | [fieldOn == 0]
  RampingUp -> peak : after(ramp, e_clk)
  peak -> RampingDown [order 2] : %check if hand is outside target
      | [inRange == 0]
  RampingDown -> minimum : after(ramp, e_clk)
  minimum -> RampingUp : %check if hand is in target and
      | %trial has a forcefield
      | [inRange == 1 && fieldOn == 1]
  (default) -> minimum
  data: ramp input double; scaling output double; tick local double; c local double; b local double; CurrScale local double; inRange input double; fieldOn input double
  events: e_clk input RISING_EDGE_EVENT
